simulink model "ds_simple_twozone"  (R2020a)
settings: Solver=ode1be  StartTime=0.0  StopTime=Inf  FixedStep=0.001  RelTol=1e-3
PostLoadFcn:
  | if any(exist('dsrtsu_mdlpostloadfcn', 'file') ~= 0), dsrtsu_mdlpostloadfcn('Execute', bdroot); end
InitFcn:
  | , if any(exist('rtifpga_mdlclblib', 'file') ~= 0), rtifpga_mdlclblib('Init', bdroot); end,
  | , if any(exist('dsmpb_private', 'file') ~= 0), dsmpb_private('dsmpb_mdlclblib', 'Init', bdroot); end,
libraries: neural x7, dsmpblib x7
(part 3 of 3)

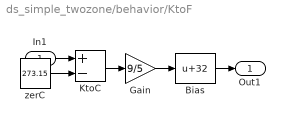
== system ds_simple_twozone/behavior/KtoF ==
  In1 : Inport
  Bias : Bias  Bias=32
  Gain : Gain  Gain=9/5
  KtoC : Sum  Inputs=+-
  zerC : Constant  Value=273.15  SampleTime=0
  Out1 : Outport
  wires:
  Gain/1 -> Bias/1
  KtoC/1 -> Gain/1
  zerC/1 -> KtoC/2
  Bias/1 -> Out1/1
  In1/1 -> KtoC/1

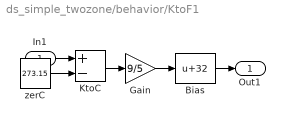
== system ds_simple_twozone/behavior/KtoF1 ==
  In1 : Inport
  Bias : Bias  Bias=32
  Gain : Gain  Gain=9/5
  KtoC : Sum  Inputs=+-
  zerC : Constant  Value=273.15  SampleTime=0
  Out1 : Outport
  wires:
  Gain/1 -> Bias/1
  KtoC/1 -> Gain/1
  zerC/1 -> KtoC/2
  Bias/1 -> Out1/1
  In1/1 -> KtoC/1

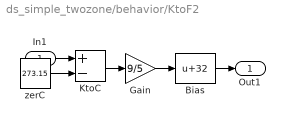
== system ds_simple_twozone/behavior/KtoF2 ==
  In1 : Inport
  Bias : Bias  Bias=32
  Gain : Gain  Gain=9/5
  KtoC : Sum  Inputs=+-
  zerC : Constant  Value=273.15  SampleTime=0
  Out1 : Outport
  wires:
  Gain/1 -> Bias/1
  KtoC/1 -> Gain/1
  zerC/1 -> KtoC/2
  Bias/1 -> Out1/1
  In1/1 -> KtoC/1

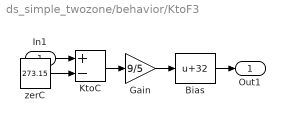
== system ds_simple_twozone/behavior/KtoF3 ==
  In1 : Inport
  Bias : Bias  Bias=32
  Gain : Gain  Gain=9/5
  KtoC : Sum  Inputs=+-
  zerC : Constant  Value=273.15  SampleTime=0
  Out1 : Outport
  wires:
  Gain/1 -> Bias/1
  KtoC/1 -> Gain/1
  zerC/1 -> KtoC/2
  Bias/1 -> Out1/1
  In1/1 -> KtoC/1

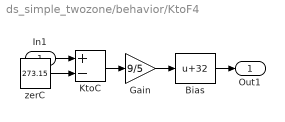
== system ds_simple_twozone/behavior/KtoF4 ==
  In1 : Inport
  Bias : Bias  Bias=32
  Gain : Gain  Gain=9/5
  KtoC : Sum  Inputs=+-
  zerC : Constant  Value=273.15  SampleTime=0
  Out1 : Outport
  wires:
  Gain/1 -> Bias/1
  KtoC/1 -> Gain/1
  zerC/1 -> KtoC/2
  Bias/1 -> Out1/1
  In1/1 -> KtoC/1

== system ds_simple_twozone/behavior/DymolaBlock/Dymola Settings ==

== system ds_simple_twozone/behavior/DymolaBlock/Modelica model2 ==

== system ds_simple_twozone/behavior/DymolaBlock/compmodel ==

== system ds_simple_twozone/behavior/DymolaBlock/editmodel ==
